simulink model "Full_scale_sim"  (R2024b)
settings: Solver=VariableStepAuto  StartTime=0.0  StopTime=60  RelTol=1e-3
values from neighbouring files (symbols this model uses):
  A_adrcl = [zeros(N, 1)  eye(N, N) ... (first row only)    [Control_Full_Scale_init_example_single_blade_installation.m]
  A_o = [A_m e_m*c_T_d_m ... (first row only)    [Control_Full_Scale_init_example_single_blade_installation.m]
  A_o_lqr = [A_m_lqr e_m*c_T_d_m_lqr ... (first row only)    [Control_Full_Scale_init_example_single_blade_installation.m]
  A_o_nmlqr = [A_m_nmlqr e_m*c_T_d_m_nmlqr ... (first row only)    [Control_Full_Scale_init_example_single_blade_installation.m]
  A_o_plqr = A_m_lqr    [Control_Full_Scale_init_example_single_blade_installation.m]
  b0 = 9.345442381739944e-04    (= 0.000934544238174)    [Control_Full_Scale_init_example_single_blade_installation.m]
  b_adrcl = [zeros(N-1, 1) ... (first row only)    [Control_Full_Scale_init_example_single_blade_installation.m]
  b_o = [b_m ... (first row only)    [Control_Full_Scale_init_example_single_blade_installation.m]
  b_o_lqr = [b_m_lqr ... (first row only)    [Control_Full_Scale_init_example_single_blade_installation.m]
  b_o_nmlqr = [b_m_nmlqr ... (first row only)    [Control_Full_Scale_init_example_single_blade_installation.m]
  b_o_plqr = b_m_lqr    [Control_Full_Scale_init_example_single_blade_installation.m]
  c_o_T = [c_T_m 0]    [Control_Full_Scale_init_example_single_blade_installation.m]
  c_o_T_lqr = [c_T_m_lqr 0]    [Control_Full_Scale_init_example_single_blade_installation.m]
  c_o_T_nmlqr = [c_T_m_nmlqr 0]    [Control_Full_Scale_init_example_single_blade_installation.m]
  c_o_T_plqr = c_T_m_lqr    [Control_Full_Scale_init_example_single_blade_installation.m]
  c_t = [1, zeros(1, N)]    [Control_Full_Scale_init_example_single_blade_installation.m]
  damping_en = 1    [Control_Full_Scale_init_example_single_blade_installation.m]
  eta_init_n = [p_init_n;Theta_init_n]    [Control_Full_Scale_init_example_single_blade_installation.m]
  k = ones(N,1)    [Control_Full_Scale_init_example_single_blade_installation.m]
  k_c_T = acker(A_m,b_m, [-omega_cl,-omega_cl])    [Control_Full_Scale_init_example_single_blade_installation.m]
  k_c_T_lqr = lqr(A_m_lqr,b_m_lqr,Q,R)    [Control_Full_Scale_init_example_single_blade_installation.m]
  k_c_T_nmlqr = lqr(A_m_nmlqr,b_m_nmlqr,Q,R)    [Control_Full_Scale_init_example_single_blade_installation.m]
  k_d_T = (e_m*c_T_d_m) \ b_m    [Control_Full_Scale_init_example_single_blade_installation.m]
  k_d_T_lqr = (e_m*c_T_d_m_lqr) \ b_m_lqr    [Control_Full_Scale_init_example_single_blade_installation.m]
  k_d_T_nmlqr = (e_m*c_T_d_m_nmlqr) \ b_m_nmlqr    [Control_Full_Scale_init_example_single_blade_installation.m]
  k_o = acker(A_o',c_o_T',[-omega_O,-omega_O,-omega_O])'    [Control_Full_Scale_init_example_single_blade_installation.m]
  k_o_lqr = acker(A_o_lqr',c_o_T_lqr',[-omega_O,-omega_O,-omega_O])'    [Control_Full_Scale_init_example_single_blade_installation.m]
  k_o_nmlqr = acker(A_o_nmlqr',c_o_T_nmlqr',[-omega_O,-omega_O,-omega_O])'    [Control_Full_Scale_init_example_single_blade_installation.m]
  k_o_plqr = acker(A_o_plqr',c_o_T_plqr',[-omega_O,-omega_O])'    [Control_Full_Scale_init_example_single_blade_installation.m]
  k_plqr = lqr(A_m_lqr, b_m_lqr, Q, R)    [Control_Full_Scale_init_example_single_blade_installation.m]
  k_s = -inv(c_T_m*inv(A_m-b_m*k_c_T)*b_m)    [Control_Full_Scale_init_example_single_blade_installation.m]
  k_s_lqr = -inv(c_T_m_lqr*inv(A_m_lqr-b_m_lqr*k_c_T_lqr)*b_m_lqr)    [Control_Full_Scale_init_example_single_blade_installation.m]
  k_s_nmlqr = -inv(c_T_m_nmlqr*inv(A_m_nmlqr-b_m_nmlqr*k_c_T_nmlqr)*b_m_nmlqr)    [Control_Full_Scale_init_example_single_blade_installation.m]
  k_s_plqr = -inv(c_T_m*inv(A_m-b_m*k_plqr)*b_m)    [Control_Full_Scale_init_example_single_blade_installation.m]
  k_w1 = gamma * EA/lw1_init    (= 68722339.2973)    [Control_Full_Scale_init_example_single_blade_installation.m]
  k_w2 = 1e8    (= 100000000)    [Control_Full_Scale_init_example_single_blade_installation.m]
  l = ones(N+1, 1)    [Control_Full_Scale_init_example_single_blade_installation.m]
  LADRC_max_effort = 900    [Control_Full_Scale_init_example_single_blade_installation.m]
  lw2 = norm(p_h_init- posSling_n(:,1))-elong_lw2    [Control_Full_Scale_init_example_single_blade_installation.m]
  meanWindSpeed = 12    [Control_Full_Scale_init_example_single_blade_installation.m]
  N = 2    [Control_Full_Scale_init_example_single_blade_installation.m]
  nu_init_b = zeros(6,1)    [Control_Full_Scale_init_example_single_blade_installation.m]
  pitch_damping = 100e+3    (= 100000)    [Control_Full_Scale_init_example_single_blade_installation.m]
  posCraneTip = [0;0;-110]    [Control_Full_Scale_init_example_single_blade_installation.m]
  posSling_b = [bladePar.posCOG + [slings_p1_new(1); -4.5; slings_p1_new(2)],                 bladePar.posCOG + [slings_p1_new(1); 4.5; slings_p1_new(2)],                bladePar.posCOG + [slings_p2_new(1); -4.5; slings_p2_new(2)],                bladePar.posCOG + [slings_p2_new(1); 4.5; slings_p2_new(2)]]    [Control_Full_Scale_init_example_single_blade_installation.m]
  posTuggerline_b = [bladePar.posCOG+[0;-4.5;0],bladePar.posCOG+[0;-35;0]]    [Control_Full_Scale_init_example_single_blade_installation.m]
undefined symbols (not defined in the file or in its folder): bladePar, k_T_d, sigbuilder_block
libraries: MarIn_blade x24, simulink_extras x3, vrlib x3, slpidlib x2, dspstat3 x1
(part 2 of 2)

== system Full_scale_sim/Thruster Assisted Single Blade Installation/Suspended blade/External force(3DOF){n} nu{b} to Force&Torque(6DOF){b}3 ==
  pos_b : Inport
  "f_ex{b} [3 X n]" : Inport  Port=2
  "eta{n}" : Inport  Port=3
  "nu{b}" : Inport  Port=4
  "Force(3DOF){b}2Force&Torque(6DOF){b}" : MarIn_blade/Basic functions/Force(3DOF){b}2Force&Torque(6DOF){b}  posCOG_bb=bladePar.posCOG
      settings: SourceProductName=MarIn(Blade)
  "pos{b} nu{b} to pos{n}" : MarIn_blade/Basic functions/pos{b} nu{b} to pos{n}  posCOG_bb=bladePar.posCOG
      settings: SourceProductName=MarIn(Blade)
  tau_ex [6n X 1] : Outport
  pos_n[3 X 1] : Outport  Port=2
  nu_n[3 X 1] : Outport  Port=3
  wires:
  "pos{b} nu{b} to pos{n}"/2 -> nu_n[3 X 1]/1
  "nu{b}"/1 -> "pos{b} nu{b} to pos{n}"/3
  "pos{b} nu{b} to pos{n}"/1 -> pos_n[3 X 1]/1
  pos_b/1 -> "Force(3DOF){b}2Force&Torque(6DOF){b}"/1, "pos{b} nu{b} to pos{n}"/1
  "Force(3DOF){b}2Force&Torque(6DOF){b}"/1 -> tau_ex [6n X 1]/1
  "f_ex{b} [3 X n]"/1 -> "Force(3DOF){b}2Force&Torque(6DOF){b}"/2
  "eta{n}"/1 -> "pos{b} nu{b} to pos{n}"/2

== system Full_scale_sim/Thruster Assisted Single Blade Installation/Suspended blade/gravity 3dof {n} ==
  mass : Inport
  Constant : Constant  Value=0
  Gain : Gain  Gain=9.81
  Mux : Mux  Inputs=3
  "gravity{n}" : Outport
  wires:
  mass/1 -> Gain/1
  Mux/1 -> "gravity{n}"/1  "Gravity"
  Constant/1 -> Mux/1, Mux/2
  Gain/1 -> Mux/3

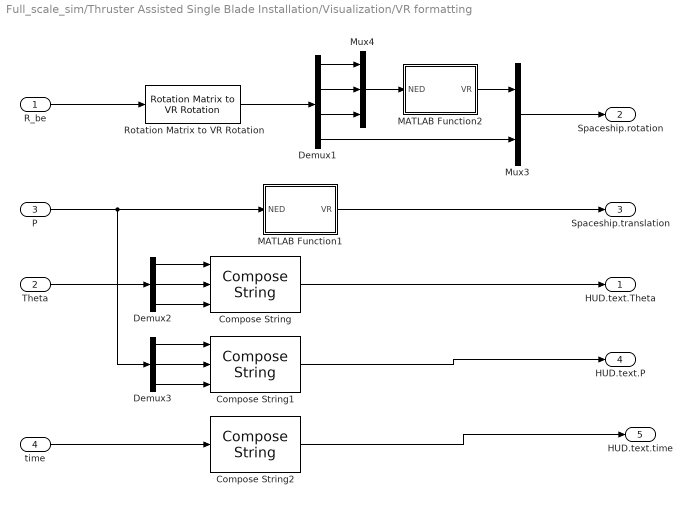
== system Full_scale_sim/Thruster Assisted Single Blade Installation/Visualization/VR formatting ==
  R_be : Inport
  Theta : Inport  Port=2
  P : Inport  Port=3
  time : Inport  Port=4
  Compose String : ComposeString  Format="'Roll    : %7.2f deg\\nPitch   : %7.2f deg\\nYaw     : %7.2f deg'"
  Compose String1 : ComposeString  Format="'X:  %7.2f m\\nY : %7.2f m\\nZ : %7.2f m'"
  Compose String2 : ComposeString  Format="'t:  %7.2f s'"
  Demux1 : Demux
  Demux2 : Demux  Outputs=3
  Demux3 : Demux  Outputs=3
  MATLAB Function1 : MATLAB Function  TreatAsAtomicUnit=on
  MATLAB Function2 : MATLAB Function  TreatAsAtomicUnit=on
  Mux3 : Mux  Inputs=2
  Mux4 : Mux  Inputs=3
  Rotation Matrix to VR Rotation : vrlib/Utilities/Rotation Matrix to VR Rotation  maxzero=1e-12
  HUD.text.Theta : Outport
  Spaceship.rotation : Outport  Port=2
  Spaceship.translation : Outport  Port=3
  HUD.text.P : Outport  Port=4
  HUD.text.time : Outport  Port=5
  wires:
  Rotation Matrix to VR Rotation/1 -> Demux1/1
  Mux3/1 -> Spaceship.rotation/1
  MATLAB Function2/1(VR) -> Mux3/1
  Mux4/1 -> MATLAB Function2/1(NED)
  Demux1/3 -> Mux4/3
  Demux1/1 -> Mux4/1
  Demux1/2 -> Mux4/2
  Demux1/4 -> Mux3/2
  MATLAB Function1/1(VR) -> Spaceship.translation/1
  Demux2/1 -> Compose String/1
  Demux2/2 -> Compose String/2
  Demux2/3 -> Compose String/3
  Compose String/1 -> HUD.text.Theta/1
  Theta/1 -> Demux2/1
  R_be/1 -> Rotation Matrix to VR Rotation/1
  Demux3/2 -> Compose String1/2
  P/1 -> Demux3/1, MATLAB Function1/1(NED)
  Demux3/3 -> Compose String1/3
  Demux3/1 -> Compose String1/1
  Compose String1/1 -> HUD.text.P/1
  time/1 -> Compose String2/1
  Compose String2/1 -> HUD.text.time/1

== matlab function Full_scale_sim/Thruster Assisted Single Blade Installation/Suspended blade/Coriolis matrix at COG  [6X6]/MATLAB Function ==
  data: tl input; coriolis6x6 output; br input
function coriolis6x6 = fcn(tl,br)
    c=zeros(6,6);
    c(1:3,1:3)=tl;
    c(4:6,4:6)=br;
coriolis6x6 = c;

== matlab function Full_scale_sim/Thruster Assisted Single Blade Installation/Visualization/VR formatting/MATLAB Function2 ==
  data: NED input; VR output
function VR = NED2VR(NED)

x = NED(1); % north
y = NED(2); % east 
z = NED(3); % down

VR = [ -y ; -z ; x ];

== matlab function Full_scale_sim/Thruster Assisted Single Blade Installation/Visualization/VR formatting/MATLAB Function1 ==
  data: NED input; VR output
function VR = NED2VR(NED)

x = NED(1); % north
y = NED(2); % east 
z = NED(3); % down

VR = [ -y ; -z ; x ];
